simulink model "lab7c"  (R2020a)
settings: Solver=VariableStepAuto  StartTime=0.0  StopTime=200  RelTol=1e-3
settings Model: Creator=ariana  LastModifiedBy=ariana

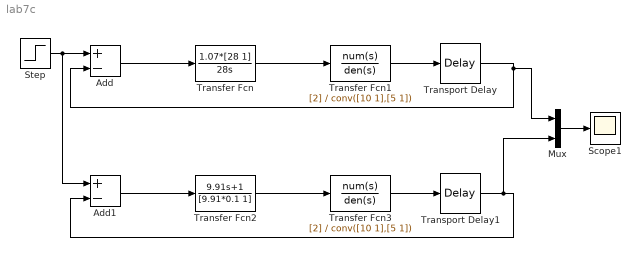
== system lab7c ==
  Add : Sum  Inputs=+-
  Add1 : Sum  Inputs=+-
  Mux : Mux  Inputs=2
  Scope1 : Scope
  Step : Step  Time=0  SampleTime=0
  Transfer Fcn : TransferFcn  Numerator=1.07*[28 1]  Denominator=[28 0]
  Transfer Fcn1 : TransferFcn  Numerator=[2]  Denominator=conv([10 1],[5 1])
  Transfer Fcn2 : TransferFcn  Numerator=[9.91 1]  Denominator=[9.91*0.1 1]
  Transfer Fcn3 : TransferFcn  Numerator=[2]  Denominator=conv([10 1],[5 1])
  Transport Delay : TransportDelay  DelayTime=3
  Transport Delay1 : TransportDelay  DelayTime=3
  wires:
  Add/1 -> Transfer Fcn/1
  Transfer Fcn/1 -> Transfer Fcn1/1
  Transfer Fcn1/1 -> Transport Delay/1
  Transport Delay/1 -> Mux/1, Add/2
  Add1/1 -> Transfer Fcn2/1
  Transfer Fcn3/1 -> Transport Delay1/1
  Transfer Fcn2/1 -> Transfer Fcn3/1
  Step/1 -> Add1/1, Add/1
  Transport Delay1/1 -> Mux/2, Add1/2
  Mux/1 -> Scope1/1
